simulink model "Modeling_of_Induction_Motor"  (R2023a)
settings: Solver=VariableStepAuto  StartTime=0.0  StopTime=15  RelTol=1e-3
libraries: spsACVoltageSourceLib x3, spsAsynchronousMachineSIUnitsLib x1, spsGroundLib x1, sps_lib x1
settings Model: SnapshotInterval=5  Creator=vande  LastModifiedBy=vande

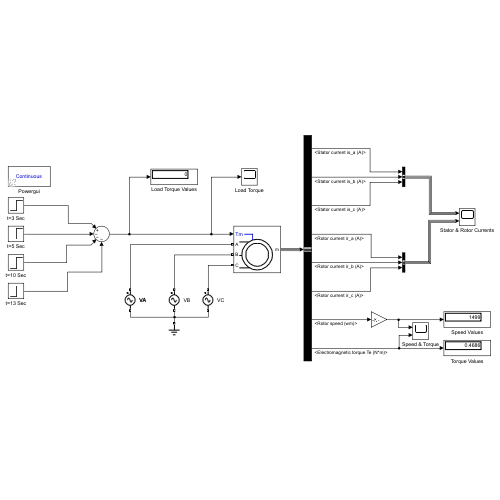
[thumbnail: Simulink's stored preview of the top-level diagram]
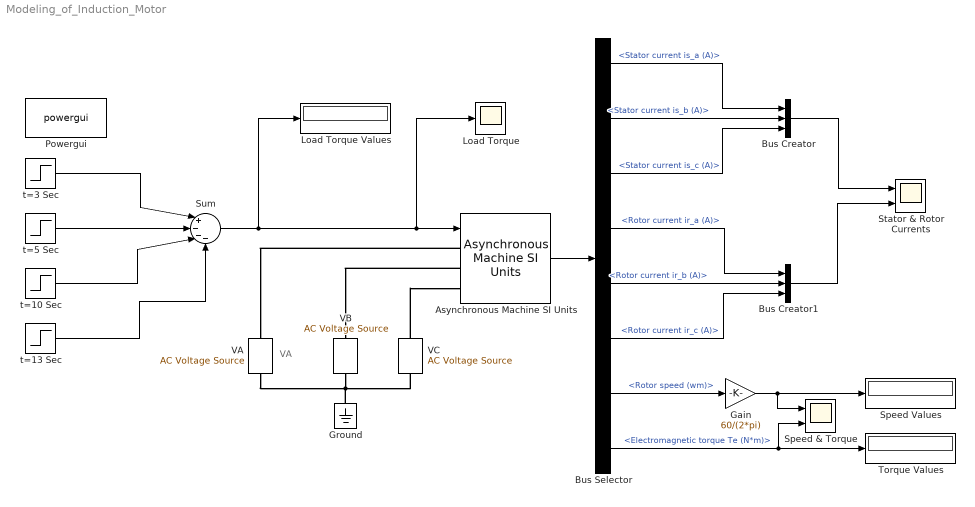
== system Modeling_of_Induction_Motor ==
  note: VA
  Asynchronous Machine SI Units : spsAsynchronousMachineSIUnitsLib/Asynchronous Machine SI Units  RotorType=Squirrel-cage  PresetModel="15:  5.4 HP (4KW)   400 V  50Hz 1430 RPM"  MechanicalLoad=Torque Tm  ShowDetailedParameters=on  ReferenceFrame=Rotor  Units=SI  MeasurementBus=off  NominalParameters=[4000 400 50]  VoltageRatio=1  Stator=[1.405 0.005839]  Rotor=[1.395 0.005839]  Cage1=[0.4155 0.002066]  Cage2=[0.4168 0.0003495]  Lm=0.1722  Mechanical=[0.0131 0.002985 2]  PolePairs=2  InitialConditions=[0 0 0 0 0 0 0 0]  SimulateSaturation=off  Saturation=[14.03593122, 27.81365428, 53.79336849, 72.68890987, 97.98006896, 148.6815601, 215.7428561, 302.9841135, 428.7778367 ; 230, 322, 414, 460, 506, 552, 598, 644, 690]  LoadFlowParameters=1492000  TsPowergui=0  TsBlock=-1  IterativeModel=Trapezoidal non iterative  IterativeDiscreteModel=Trapezoidal non iterative  Pmec=1.492e+006
  Bus Creator : BusCreator  Inputs=3
  Bus Creator1 : BusCreator  Inputs=3
  Bus Selector : BusSelector  OutputSignals=Stator measurements.Stator current is_a (A),Stator measurements.Stator current is_b (A),Stator measurements.Stator current is_c (A),Rotor measurements.Rotor current ir_a (A),Rotor measurements.Rotor current ir_b (A),Rotor measurements.Rotor current ir_c (A),Mechanical.Rotor speed (wm),Mechanical.Electromagnetic torque Te (N*m)
  Gain : Gain  Gain=60/(2*pi)
  Ground : spsGroundLib/Ground  LConnTagsString=a
  Load Torque : Scope
  Load Torque Values : Display
  Powergui : sps_lib/powergui  Priority=1  SimulationMode=Continuous  SampleTime=50e-6  frequency=60  Iterations=50  frequencyindice=50  Pbase=100e6  ErrMax=1e-4  UnitsV=kV  UnitsW=MW  buscounter=0  FunctionMessages=off  echomessages=off  EnableUseOfTLC=off  CurrentSourceSwitches=off  DisableSnubberDevices=off  DisableRonSwitches=off  DisableVfSwitches=off  DisplayEquations=off  AutomaticDiscreteSolvers=off  SolverType=Tustin/Backward Euler (TBE)  Interpol=off  ExternalGateDelay=off  methode=off  Ts=100  x0status=blocks  SPID=on  SwTol=0  HookPort=off  NonlinearTolerance=1e-4  nMaxIteration=100  ContinueOnMaxIteration=off  RestoreLinks=warning  ResistiveCurrentMeasurement=off  Frange=[0:2:500]  Ylog=off  Xlog=on  ShowGrid=off  save=off  variable=ZData  structure=0  ZoomFFT=off  StartTime=0.0  cycles=1  DisplayStyle=1  fundamental=60  FreqAxis=off  MaxFrequency=1000  frequencyindicesteady=1  RmsSteady=1  display=off
  Speed & Torque : Scope  NumInputPorts=2
  Speed Values : Display
  Stator & Rotor Currents : Scope  NumInputPorts=2
  Sum : Sum  Inputs=|+---
  Torque Values : Display
  VA : spsACVoltageSourceLib/AC Voltage Source  Amplitude=326.54  Phase=0  Frequency=50  SampleTime=0  Measurements=None  BusType=swing  Pref=10e3  Qref=0  Qmin=-inf  Qmax=+inf
  VB : spsACVoltageSourceLib/AC Voltage Source  Amplitude=326.54  Phase=-120  Frequency=50  SampleTime=0  Measurements=None  BusType=swing  Pref=10e3  Qref=0  Qmin=-inf  Qmax=+inf
  VC : spsACVoltageSourceLib/AC Voltage Source  Amplitude=326.54  Phase=120  Frequency=50  SampleTime=0  Measurements=None  BusType=swing  Pref=10e3  Qref=0  Qmin=-inf  Qmax=+inf
  t=10 Sec : Step  Time=10  After=6.68  SampleTime=0
  t=13 Sec : Step  Time=13  After=6.68  SampleTime=0
  t=3 Sec : Step  Time=3  After=26.72  SampleTime=0
  t=5 Sec : Step  Time=5  After=13.36  SampleTime=0
  wires:
  t=3 Sec/1 -> Sum/1
  t=5 Sec/1 -> Sum/2
  t=10 Sec/1 -> Sum/3
  Bus Selector/7 -> Gain/1  "<Rotor speed (wm)>"
  Sum/1 -> Asynchronous Machine SI Units/1, Load Torque/1, Load Torque Values/1
  t=13 Sec/1 -> Sum/4
  Bus Selector/8 -> Torque Values/1, Speed & Torque/2  "<Electromagnetic torque Te (N*m)>"
  Asynchronous Machine SI Units/1 -> Bus Selector/1
  Gain/1 -> Speed Values/1, Speed & Torque/1
  Bus Selector/4 -> Bus Creator1/1  "<Rotor current ir_a (A)>"
  Bus Selector/5 -> Bus Creator1/2  "<Rotor current ir_b (A)>"
  Bus Selector/1 -> Bus Creator/1  "<Stator current is_a (A)>"
  Bus Selector/2 -> Bus Creator/2  "<Stator current is_b (A)>"
  Bus Selector/3 -> Bus Creator/3  "<Stator current is_c (A)>"
  Bus Selector/6 -> Bus Creator1/3  "<Rotor current ir_c (A)>"
  Bus Creator1/1 -> Stator & Rotor Currents/2
  Bus Creator/1 -> Stator & Rotor Currents/1
  connections:
  Asynchronous Machine SI Units/LConn1 -- VA/RConn1
  Asynchronous Machine SI Units/LConn2 -- VB/RConn1
  VA/LConn1 -- Ground/LConn1 -- VB/LConn1 -- VC/LConn1
  VC/RConn1 -- Asynchronous Machine SI Units/LConn3
